simulink model "direct_graph_2D_TBG_spanning_tree"  (R2020a)
settings: Solver=FixedStepAuto  StartTime=0.0  StopTime=10.0  FixedStep=0.0001  RelTol=1e-3
settings Model: Creator=WangQipeng  LastModifiedBy=WangQipeng

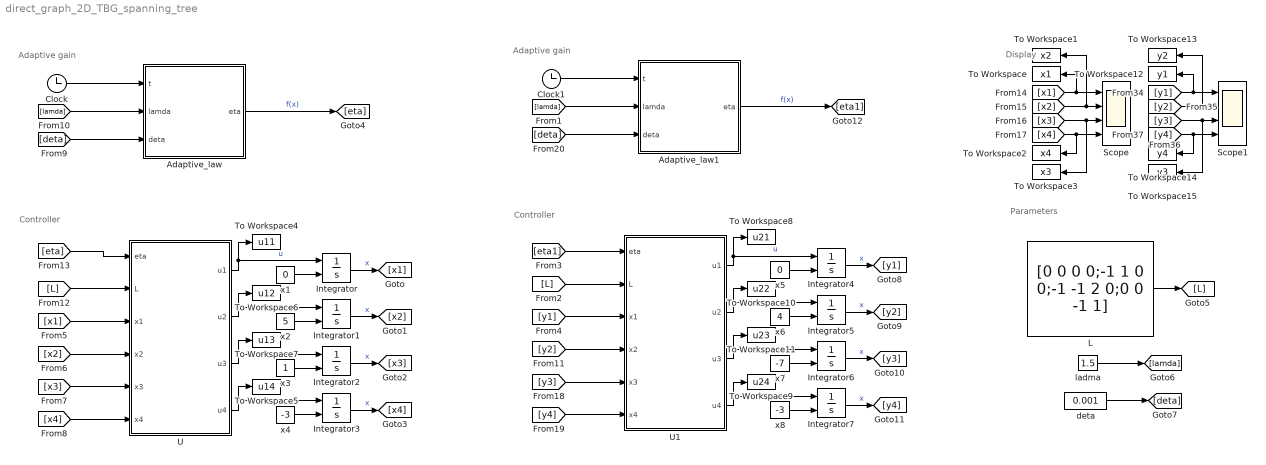
== system direct_graph_2D_TBG_spanning_tree ==
  note: Controller
  note: Adaptive gain
  note: Parameters
  note: Adaptive gain
  note: Controller
  note: Display
  Adaptive_law : MATLAB Function  TreatAsAtomicUnit=on
  Adaptive_law1 : MATLAB Function  TreatAsAtomicUnit=on
  Clock : Clock
  Clock1 : Clock
  Integrator{,1..7} (8 alike) : Integrator  InitialConditionSource=external  InitialCondition=1
  L : Constant  Value=[0 0 0 0;-1 1 0 0;-1 -1 2 0;0 0 -1 1]
  Scope : Scope  NumInputPorts=4
  Scope1 : Scope  NumInputPorts=4
  To Workspace : ToWorkspace  VariableName=x1  SaveFormat=Timeseries  SampleTime=-1
  To Workspace1 : ToWorkspace  VariableName=x2  SaveFormat=Timeseries  SampleTime=-1
  To Workspace10 : ToWorkspace  VariableName=u22  SaveFormat=Timeseries  SampleTime=-1
  To Workspace11 : ToWorkspace  VariableName=u23  SaveFormat=Timeseries  SampleTime=-1
  To Workspace12 : ToWorkspace  VariableName=y1  SaveFormat=Timeseries  SampleTime=-1
  To Workspace13 : ToWorkspace  VariableName=y2  SaveFormat=Timeseries  SampleTime=-1
  To Workspace14 : ToWorkspace  VariableName=y4  SaveFormat=Timeseries  SampleTime=-1
  To Workspace15 : ToWorkspace  VariableName=y3  SaveFormat=Timeseries  SampleTime=-1
  To Workspace2 : ToWorkspace  VariableName=x4  SaveFormat=Timeseries  SampleTime=-1
  To Workspace3 : ToWorkspace  VariableName=x3  SaveFormat=Timeseries  SampleTime=-1
  To Workspace4 : ToWorkspace  VariableName=u11  SaveFormat=Timeseries  SampleTime=-1
  To Workspace5 : ToWorkspace  VariableName=u14  SaveFormat=Timeseries  SampleTime=-1
  To Workspace6 : ToWorkspace  VariableName=u12  SaveFormat=Timeseries  SampleTime=-1
  To Workspace7 : ToWorkspace  VariableName=u13  SaveFormat=Timeseries  SampleTime=-1
  To Workspace8 : ToWorkspace  VariableName=u21  SaveFormat=Timeseries  SampleTime=-1
  To Workspace9 : ToWorkspace  VariableName=u24  SaveFormat=Timeseries  SampleTime=-1
  U : MATLAB Function  TreatAsAtomicUnit=on
  U1 : MATLAB Function  TreatAsAtomicUnit=on
  deta : Constant  Value=0.001
  ladma : Constant  Value=1.5
  x1 : Constant  Value=0
  x2 : Constant  Value=5
  x3 : Constant
  x4 : Constant  Value=-3
  x5 : Constant  Value=0
  x6 : Constant  Value=4
  x7 : Constant  Value=-7
  x8 : Constant  Value=-3
  wires:
  U/1(u1) -> To Workspace4/1, Integrator/1  "u"
  U/2(u2) -> To Workspace6/1, Integrator1/1
  U/3(u3) -> To Workspace7/1, Integrator2/1
  U/4(u4) -> Integrator3/1, To Workspace5/1
  Integrator/1 -> [x1]  "x"
  Integrator1/1 -> [x2]  "x"
  Integrator2/1 -> [x3]  "x"
  Integrator3/1 -> [x4]  "x"
  [x3] -> U/5(x3)
  [x4] -> U/6(x4)
  [x1] -> U/3(x1)
  [x2] -> U/4(x2)
  L/1 -> [L]
  [deta] -> Adaptive_law/3(deta)
  ladma/1 -> [lamda]
  deta/1 -> [deta]
  [lamda] -> Adaptive_law/2(lamda)
  Clock/1 -> Adaptive_law/1(t)
  [L] -> U/2(L)
  [eta] -> U/1(eta)
  x1/1 -> Integrator/2
  x2/1 -> Integrator1/2
  x3/1 -> Integrator2/2
  x4/1 -> Integrator3/2
  Adaptive_law/1(eta) -> [eta]  "f(x)"
  Adaptive_law1/1(eta) -> [eta1]  "f(x)"
  [y2] -> U1/4(x2)
  [y3] -> U1/5(x3)
  x5/1 -> Integrator4/2
  x8/1 -> Integrator7/2
  x7/1 -> Integrator6/2
  [deta] -> Adaptive_law1/3(deta)
  Integrator7/1 -> [y4]  "x"
  [eta1] -> U1/1(eta)
  Clock1/1 -> Adaptive_law1/1(t)
  U1/3(u3) -> To Workspace11/1, Integrator6/1
  [y4] -> U1/6(x4)
  [y1] -> U1/3(x1)
  x6/1 -> Integrator5/2
  [L] -> U1/2(L)
  Integrator5/1 -> [y2]  "x"
  U1/2(u2) -> To Workspace10/1, Integrator5/1
  U1/4(u4) -> Integrator7/1, To Workspace9/1
  U1/1(u1) -> To Workspace8/1, Integrator4/1  "u"
  Integrator6/1 -> [y3]  "x"
  [lamda] -> Adaptive_law1/2(lamda)
  Integrator4/1 -> [y1]  "x"
  [y3] -> Scope1/3, To Workspace15/1
  [x3] -> Scope/3, To Workspace3/1
  [x4] -> Scope/4, To Workspace2/1
  [x1] -> Scope/1, To Workspace/1
  [y2] -> To Workspace13/1, Scope1/2
  [x2] -> To Workspace1/1, Scope/2
  [y1] -> Scope1/1, To Workspace12/1
  [y4] -> Scope1/4, To Workspace14/1

== matlab function direct_graph_2D_TBG_spanning_tree/U ==
  data: eta input; u1 output; L input; x1 input; x2 input; x3 input; x4 input; u2 output; u3 output; u4 output
function [u1,u2,u3,u4] = protocol(eta,L,x1,x2,x3,x4)
x = [x1;x2;x3;x4];
temp = -(eta + 1) * L * x;

%temp_u1 = temp(1);
u1 = 0;
u2 = temp(2);
u3 = temp(3);
u4 = temp(4);

== matlab function direct_graph_2D_TBG_spanning_tree/Adaptive_law ==
  data: t input; eta output; lamda input; deta input
function eta = TBG(t,lamda,deta)
%%%%%%% h=[2;1;1]   %%%%%%%%%%
if(t<=4)
    zeta = 10/(4^6)*t^6 - 24/(4^5)*t^5 + 15/(4^4)*t^4;
    d_zeta = 60/(4^6)*t^5 - 120/(4^5)*t^4 + 15/(4^3)*t^3;
else
    zeta = 1;
    d_zeta = 0;
end

eta = 2*d_zeta/(lamda * (1 - zeta + deta));

== matlab function direct_graph_2D_TBG_spanning_tree/Adaptive_law1 ==
  data: t input; eta output; lamda input; deta input
function eta = TBG(t,lamda,deta)
%%%%%%% h=[2;1;1]   %%%%%%%%%%
if(t<=4)
    zeta = 10/(4^6)*t^6 - 24/(4^5)*t^5 + 15/(4^4)*t^4;
    d_zeta = 60/(4^6)*t^5 - 120/(4^5)*t^4 + 15/(4^3)*t^3;
else
    zeta = 1;
    d_zeta = 0;
end

eta = 2*d_zeta/(lamda * (1 - zeta + deta));

== matlab function direct_graph_2D_TBG_spanning_tree/U1 ==
  data: eta input; u1 output; L input; x1 input; x2 input; x3 input; x4 input; u2 output; u3 output; u4 output
function [u1,u2,u3,u4] = protocol(eta,L,x1,x2,x3,x4)
x = [x1;x2;x3;x4];
temp = -(eta + 1) * L * x;

%temp_u1 = temp(1);
u1 = 0;
u2 = temp(2);
u3 = temp(3);
u4 = temp(4);
